simulink model "simulacao2"  (R2018a)
settings: Solver=VariableStepAuto  StartTime=0.0  StopTime=50000  RelTol=1e-3
settings Model: Creator=Christopher  LastModifiedBy=Christopher

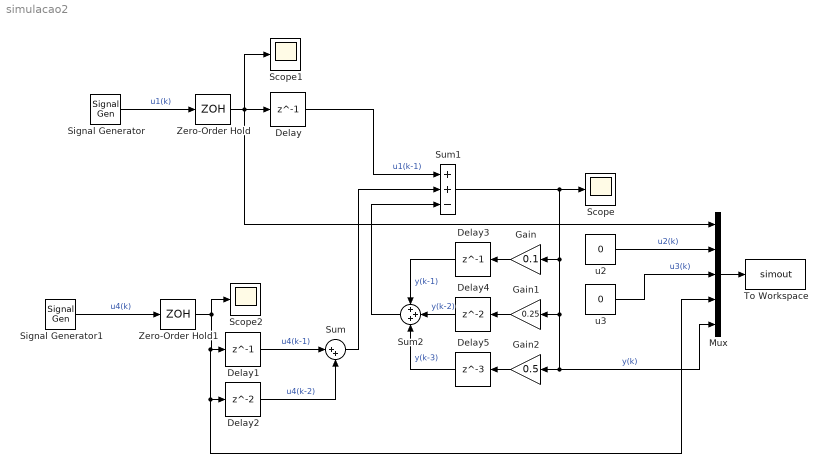
== system simulacao2 ==
  Delay : Delay  DelayLength=1
  Delay1 : Delay  DelayLength=1
  Delay2 : Delay
  Delay3 : Delay  DelayLength=1
  Delay4 : Delay
  Delay5 : Delay  DelayLength=3
  Gain : Gain  Gain=0.1
  Gain1 : Gain  Gain=0.25
  Gain2 : Gain  Gain=0.5
  Mux : Mux  Inputs=5
  Scope : Scope
  Scope1 : Scope
  Scope2 : Scope
  Signal Generator : SignalGenerator  WaveForm=random  Units=rad/sec
  Signal Generator1 : SignalGenerator  WaveForm=random  Units=rad/sec
  Sum : Sum  Inputs=|++
  Sum1 : Sum  Inputs=++-
  Sum2 : Sum  Inputs=+++
  To Workspace : ToWorkspace  VariableName=simout  SampleTime=-1
  Zero-Order Hold : ZeroOrderHold
  Zero-Order Hold1 : ZeroOrderHold
  u2 : Constant  Value=0  SampleTime=1
  u3 : Constant  Value=0  SampleTime=1
  wires:
  Delay1/1 -> Sum/1  "u4(k-1)"
  Delay2/1 -> Sum/2  "u4(k-2)"
  Delay/1 -> Sum1/1  "u1(k-1)"
  Sum/1 -> Sum1/2
  Sum1/1 -> Scope/1, Mux/5, Gain2/1, Gain1/1, Gain/1  "y(k)"
  Delay3/1 -> Sum2/1  "y(k-1)"
  Delay4/1 -> Sum2/2  "y(k-2)"
  Delay5/1 -> Sum2/3  "y(k-3)"
  Sum2/1 -> Sum1/3
  Mux/1 -> To Workspace/1
  u2/1 -> Mux/2  "u2(k)"
  u3/1 -> Mux/3  "u3(k)"
  Signal Generator/1 -> Zero-Order Hold/1  "u1(k)"
  Signal Generator1/1 -> Zero-Order Hold1/1  "u4(k)"
  Gain/1 -> Delay3/1
  Gain1/1 -> Delay4/1
  Gain2/1 -> Delay5/1
  Zero-Order Hold/1 -> Mux/1, Delay/1, Scope1/1
  Zero-Order Hold1/1 -> Scope2/1, Mux/4, Delay2/1, Delay1/1
